simulink model "CascadeFFW"  (R2020a)
settings: Solver=VariableStepAuto  StartTime=0.0  StopTime=15  RelTol=1e-3
values from neighbouring files (symbols this model uses):
  gain_P = ControlSystemDesignerSession.DesignerData.Designs.Data.C.K    [script_cascade.m]
  gain_V_I = gains_PI(2)    [script_cascade.m]
  gain_V_P = gains_PI(1)    [script_cascade.m]
settings Model: Creator=Admin  LastModifiedBy=Admin
settings DataIOCC: ReturnWorkspaceOutputsName=out_ffw

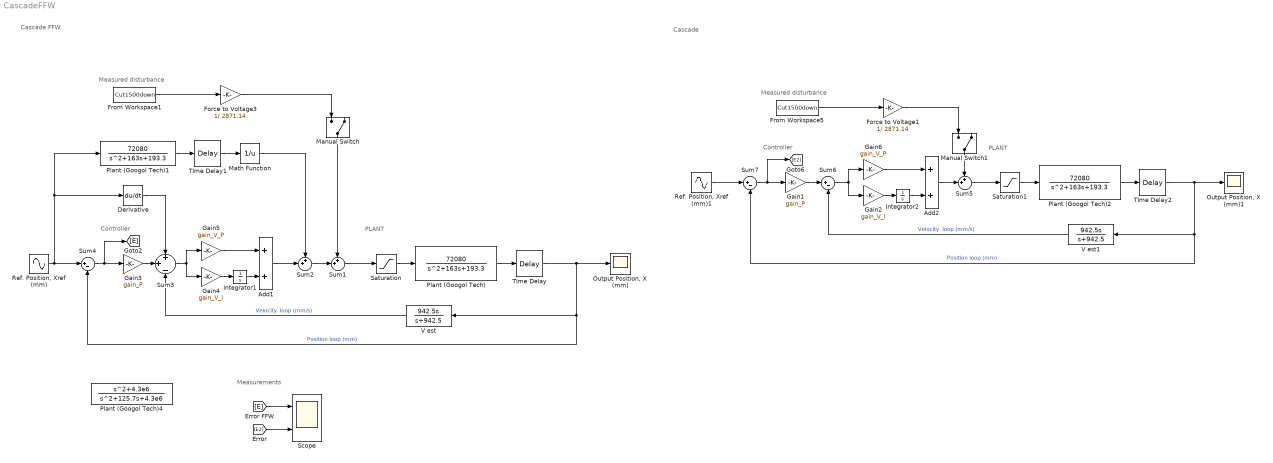
== system CascadeFFW ==
  note: Measurements
  note: Cascade FFW
  note: Controller
  note: PLANT
  note: Measured disturbance
  note: Cascade
  note: Controller
  note: PLANT
  note: Measured disturbance
  Add1 : Sum
  Add2 : Sum
  Derivative : Derivative
  Force to Voltage1 : Gain  Gain=1/ 2871.14
  Force to Voltage3 : Gain  Gain=1/ 2871.14
  From Workspace1 : FromWorkspace  VariableName=Cut1500down  OutDataTypeStr=double  OutputAfterFinalValue=Setting to zero
  From Workspace5 : FromWorkspace  VariableName=Cut1500down  OutDataTypeStr=double  OutputAfterFinalValue=Setting to zero
  Gain1 : Gain  Gain=gain_P
  Gain2 : Gain  Gain=gain_V_I
  Gain3 : Gain  Gain=gain_P
  Gain4 : Gain  Gain=gain_V_I
  Gain5 : Gain  Gain=gain_V_P
  Gain6 : Gain  Gain=gain_V_P
  Integrator1 : Integrator  InitialCondition=.1
  Integrator2 : Integrator  InitialCondition=.1
  Manual Switch : ManualSwitch  CurrentSetting=0
  Manual Switch1 : ManualSwitch  CurrentSetting=0
  Math Function : Math  Operator=reciprocal  SaturateOnIntegerOverflow=on
  "Output Position, X (mm)" : Scope
  "Output Position, X (mm)1" : Scope
  Plant (Googol Tech) : TransferFcn  Numerator=[72080]  Denominator=[1 163 193.3]
  Plant (Googol Tech)1 : TransferFcn  Numerator=[72080]  Denominator=[1 163 193.3]
  Plant (Googol Tech)2 : TransferFcn  Numerator=[72080]  Denominator=[1 163 193.3]
  Plant (Googol Tech)4 : TransferFcn  Numerator=[1 0 4.3e6]  Denominator=[1 125.7 4.3e6]
  "Ref. Position, Xref (mm)" : Sin  Amplitude=5  Frequency=0.5*(2*pi)  SampleTime=0  Offset=1/2000
  "Ref. Position, Xref (mm)1" : Sin  Amplitude=5  Frequency=0.5*(2*pi)  SampleTime=0  Offset=1/2000
  Saturation : Saturate  UpperLimit=92  LowerLimit=-92
  Saturation1 : Saturate  UpperLimit=92  LowerLimit=-92
  Scope : Scope  NumInputPorts=2
  Sum1 : Sum  Inputs=++|
  Sum2 : Sum  Inputs=++|
  Sum3 : Sum  Inputs=+|+|-
  Sum4 : Sum  Inputs=|+-
  Sum5 : Sum  Inputs=++|
  Sum6 : Sum  Inputs=|+-
  Sum7 : Sum  Inputs=|+-
  TIme Delay : TransportDelay  DelayTime=0.0012
  TIme Delay1 : TransportDelay  DelayTime=0.0012
  TIme Delay2 : TransportDelay  DelayTime=0.0012
  V est : TransferFcn  Numerator=[942.5, 0]  Denominator=[1 942.5]
  V est1 : TransferFcn  Numerator=[942.5, 0]  Denominator=[1 942.5]
  wires:
  TIme Delay/1 -> "Output Position, X (mm)"/1, V est/1, Sum4/2  "Position loop (mm)"
  Integrator1/1 -> Add1/2
  Manual Switch/1 -> Sum1/1
  Gain3/1 -> Sum3/2
  "Ref. Position, Xref (mm)"/1 -> Plant (Googol Tech)1/1, Derivative/1, Sum4/1
  [E2] -> Scope/2
  Sum3/1 -> Gain4/1, Gain5/1
  Sum1/1 -> Saturation/1
  Add1/1 -> Sum2/2
  Sum4/1 -> Gain3/1, [E]
  [E] -> Scope/1
  Plant (Googol Tech)/1 -> TIme Delay/1
  V est/1 -> Sum3/3  "Velocity  loop (mm/s)"
  Gain4/1 -> Integrator1/1
  Saturation/1 -> Plant (Googol Tech)/1
  Gain5/1 -> Add1/1
  Derivative/1 -> Sum3/1
  Sum2/1 -> Sum1/2
  Plant (Googol Tech)1/1 -> TIme Delay1/1
  TIme Delay1/1 -> Math Function/1
  Math Function/1 -> Sum2/1
  TIme Delay2/1 -> "Output Position, X (mm)1"/1, Sum7/2, V est1/1  "Position loop (mm)"
  From Workspace5/1 -> Force to Voltage1/1
  Integrator2/1 -> Add2/2
  Manual Switch1/1 -> Sum5/1
  Gain1/1 -> Sum6/1
  "Ref. Position, Xref (mm)1"/1 -> Sum7/1
  Sum6/1 -> Gain6/1, Gain2/1
  Sum5/1 -> Saturation1/1
  Add2/1 -> Sum5/2
  Sum7/1 -> Gain1/1, [E2]
  Plant (Googol Tech)2/1 -> TIme Delay2/1
  V est1/1 -> Sum6/2  "Velocity  loop (mm/s)"
  Gain2/1 -> Integrator2/1
  Saturation1/1 -> Plant (Googol Tech)2/1
  Gain6/1 -> Add2/1
  Force to Voltage1/1 -> Manual Switch1/1
  From Workspace1/1 -> Force to Voltage3/1
  Force to Voltage3/1 -> Manual Switch/1
